simulink model "etb_positionControlModel"  (R2019b)
settings: Solver=FixedStepAuto  StartTime=0.0  StopTime=2  FixedStep=.001  RelTol=1e-3
values from neighbouring files (symbols this model uses):
  motorPosCmd = 60    [etb_positionControlModelSweep.m]
  motorPosGainI = 0    [etb_positionControlModelSweep.m]
  motorPosGainP = 1000:500:2500    [etb_positionControlModelSweep.m]
  motorVelGainFeedback = 200    [etb_positionControlModelSweep.m]
  motorVelGainI = 2500    [etb_positionControlModelSweep.m]
  motorVelGainP = 200:200:1000    [etb_positionControlModelSweep.m]
  springConst = 200    [etb_positionControlModelSweep.m]    (also in sweepSpringConstant.m = 300; sweepSpringFullSweep.m = 300; sweepSpringFullSweep_Ron.m = 300; sweepSpringPreload.m = 300)
  springPreload = 800    [etb_positionControlModelSweep.m]    (also in sweepSpringConstant.m = 780; sweepSpringFullSweep.m = 780; sweepSpringFullSweep_Ron.m = 780; sweepSpringPreload.m = 780)
undefined symbols (not defined in the file or in its folder): DiscIntNeverNeededParam
libraries: simulink x3, eeGeneralControl x1
settings Model: Creator=Nick  LastModifiedBy=Nick

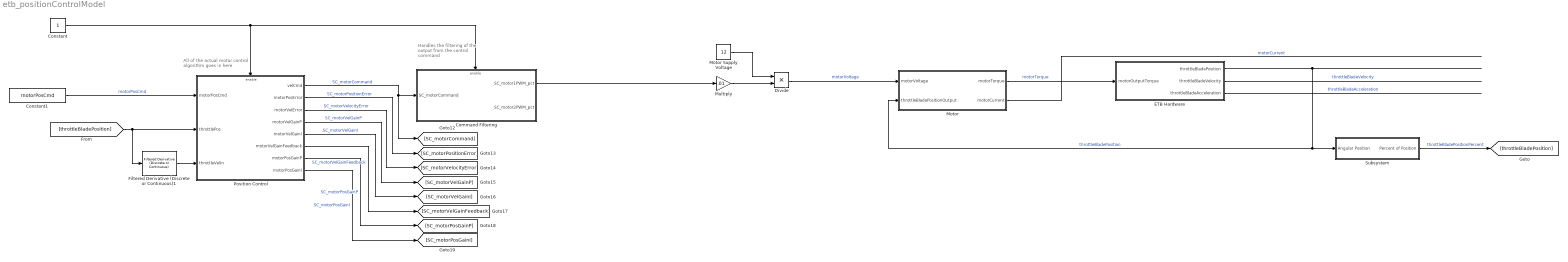
== system etb_positionControlModel ==
  note: All of the actual motor control algorithm goes in here
  note: Handles the filtering of the output from the control command
  Command Filtering : Subsystem
  Constant : Constant
  Constant1 : Constant  Value=motorPosCmd
  Divide : Product  Inputs=**
  ETB Hardware : Subsystem
  Filtered Derivative (Discrete or Continuous)1 : eeGeneralControl/Filtered Derivative (Discrete or Continuous)  K=1  T=0.01  B=inf  A=-inf  minRatio=10  Ts=-1
      settings: SourceProductName=Simscape Electrical  SourceProductBaseCode=PS
  Motor : Subsystem
  Motor Supply Voltage : Constant  Value=12
  Multiply : Gain  Gain=.01
  Position Control : Subsystem  TreatAsAtomicUnit=on
  Subsystem : Subsystem
  wires:
  ETB Hardware/2(throttleBladeVelocity) -> ?  "throttleBladeVelocity"
  ETB Hardware/3(throttleBladeAcceleration) -> ?  "throttleBladeAcceleration"
  Motor/1(motorTorque) -> ETB Hardware/1(motorOutputTorque)  "motorTorque"
  Motor/2(motorCurrent) -> ?  "motorCurrent"
  ETB Hardware/1(throttleBladePosition) -> Subsystem/1(Angular Position), Motor/2(throttleBladePositionOutput)  "throttleBladePosition"
  Divide/1 -> Motor/1(motorVoltage)  "motorVoltage"
  Multiply/1 -> Divide/2
  Motor Supply Voltage/1 -> Divide/1
  Command Filtering/1(SC_motor1PWM_pct) -> Multiply/1
  Subsystem/1(Percent of Position) -> [throttleBladePosition]  "throttleBladePositionPercent"
  [throttleBladePosition] -> Filtered Derivative (Discrete or Continuous)1/1, Position Control/2(throttlePos)
  Constant1/1 -> Position Control/1(motorPosCmd)  "motorPosCmd"
  Filtered Derivative (Discrete or Continuous)1/1 -> Position Control/3(throttleVelIn)
  Constant/1 -> Position Control/Enable, Command Filtering/Enable
  Position Control/1(velCmd) -> Command Filtering/1(SC_motorCommand), [SC_motorCommand]  "SC_motorCommand"
  Position Control/5(motorVelGainI) -> [SC_motorVelGainI]  "SC_motorVelGainI"
  Position Control/3(motorVelError) -> [SC_motorVelocityError]  "SC_motorVelocityError"
  Position Control/7(motorPosGainP) -> [SC_motorPosGainP]  "SC_motorPosGainP"
  Position Control/6(motorVelGainFeedback) -> [SC_motorVelGainFeedback]  "SC_motorVelGainFeedback"
  Position Control/4(motorVelGainP) -> [SC_motorVelGainP]  "SC_motorVelGainP"
  Position Control/2(motorPosError) -> [SC_motorPositionError]  "SC_motorPositionError"
  Position Control/8(motorPosGainI) -> [SC_motorPosGainI]  "SC_motorPosGainI"

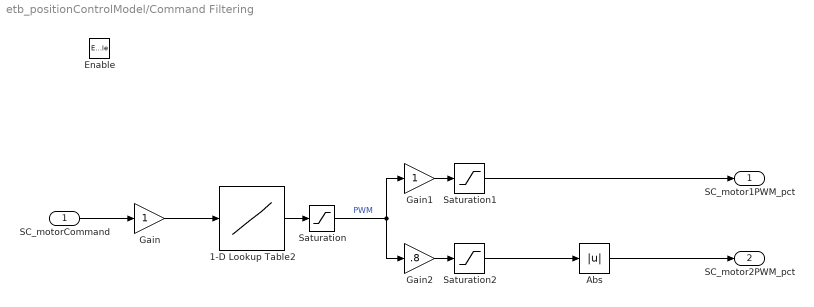
== system etb_positionControlModel/Command Filtering ==
  SC_motorCommand : Inport
  Enable : EnablePort  StatesWhenEnabling=reset
  1-D Lookup Table2 : Lookup_n-D  NumberOfTableDimensions=1  BreakpointsForDimension1=[-100 -5 -.1 0 .1 5 100]  Table=[-100 -5 -1 0 1 20 100]  InternalRulePriority=Speed  RndMeth=Simplest  InputSameDT=on
  Abs : Abs
  Gain : Gain
  Gain1 : Gain
  Gain2 : Gain  Gain=.8
  Saturation : Saturate  UpperLimit=100  LowerLimit=-100
  Saturation1 : Saturate  UpperLimit=100  LowerLimit=0
  Saturation2 : Saturate  UpperLimit=0  LowerLimit=-100
  SC_motor1PWM_pct : Outport
  SC_motor2PWM_pct : Outport  Port=2
  wires:
  Abs/1 -> SC_motor2PWM_pct/1
  1-D Lookup Table2/1 -> Saturation/1
  Gain/1 -> 1-D Lookup Table2/1
  Saturation2/1 -> Abs/1
  Gain1/1 -> Saturation1/1
  Gain2/1 -> Saturation2/1
  SC_motorCommand/1 -> Gain/1
  Saturation/1 -> Gain1/1, Gain2/1  "PWM"
  Saturation1/1 -> SC_motor1PWM_pct/1

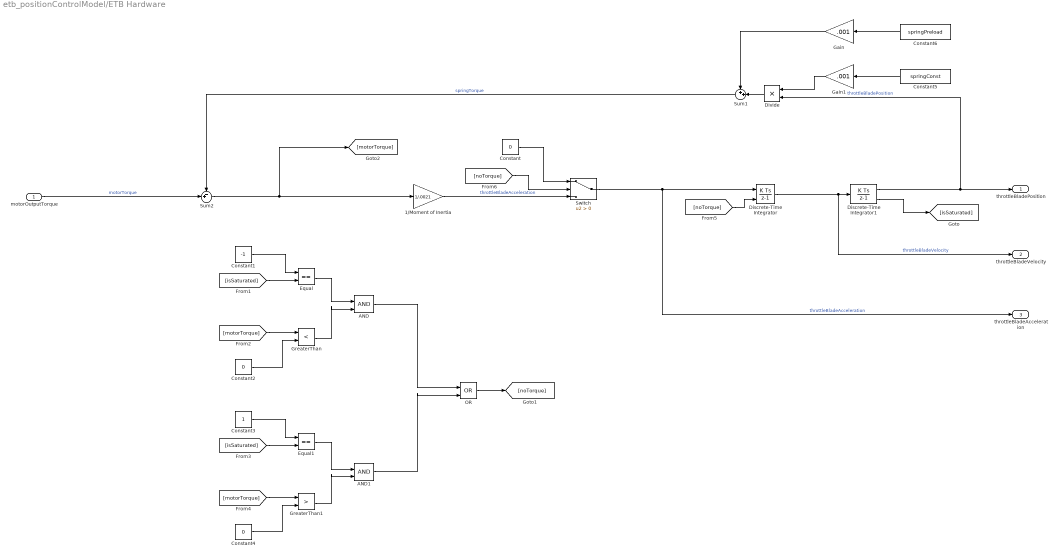
== system etb_positionControlModel/ETB Hardware ==
  motorOutputTorque : Inport
  1/Moment of Inertia : Gain  Gain=1/.0021
  AND : Logic  IconShape=distinctive  AllPortsSameDT=off  OutDataTypeStr=boolean
  AND1 : Logic  IconShape=distinctive  AllPortsSameDT=off  OutDataTypeStr=boolean
  Constant : Constant  Value=0
  Constant1 : Constant  Value=-1
  Constant2 : Constant  Value=0
  Constant3 : Constant
  Constant4 : Constant  Value=0
  Constant5 : Constant  Value=springConst
  Constant6 : Constant  Value=springPreload
  Discrete-Time Integrator : DiscreteIntegrator  ExternalReset=level  SampleTime=-1  ICPrevOutput=DiscIntNeverNeededParam  ICPrevScaledInput=DiscIntNeverNeededParam
  Discrete-Time Integrator1 : DiscreteIntegrator  SampleTime=-1  LimitOutput=on  UpperSaturationLimit=1.5708  LowerSaturationLimit=0  ShowSaturationPort=on  ICPrevOutput=DiscIntNeverNeededParam  ICPrevScaledInput=DiscIntNeverNeededParam
  Divide : Product  Inputs=**
  Equal : RelationalOperator  Operator===  OutDataTypeStr=boolean  RndMeth=Simplest
  Equal1 : RelationalOperator  Operator===  OutDataTypeStr=boolean  RndMeth=Simplest
  Gain : Gain  Gain=.001
  Gain1 : Gain  Gain=.001
  GreaterThan : RelationalOperator  Operator=<  OutDataTypeStr=boolean  RndMeth=Simplest
  GreaterThan1 : RelationalOperator  Operator=>  OutDataTypeStr=boolean  RndMeth=Simplest
  OR : Logic  Operator=OR  IconShape=distinctive  AllPortsSameDT=off  OutDataTypeStr=boolean
  Sum1 : Sum  Inputs=++|
  Sum2 : Sum  Inputs=-+|
  Switch : Switch  Criteria=u2 > Threshold
  throttleBladePosition : Outport
  throttleBladeVelocity : Outport  Port=2
  throttleBladeAcceleration : Outport  Port=3
  wires:
  Constant5/1 -> Gain1/1
  Gain1/1 -> Divide/1
  Constant6/1 -> Gain/1
  motorOutputTorque/1 -> Sum2/2  "motorTorque"
  Sum1/1 -> Sum2/1  "springTorque"
  Switch/1 -> Discrete-Time Integrator/1, throttleBladeAcceleration/1  "throttleBladeAcceleration"
  Discrete-Time Integrator/1 -> throttleBladeVelocity/1, Discrete-Time Integrator1/1  "throttleBladeVelocity"
  Discrete-Time Integrator1/1 -> throttleBladePosition/1, Divide/2  "throttleBladePosition"
  Divide/1 -> Sum1/2
  Gain/1 -> Sum1/1
  Sum2/1 -> 1/Moment of Inertia/1, [motorTorque]
  Constant1/1 -> Equal/1
  Equal/1 -> AND/1
  Discrete-Time Integrator1/2 -> [isSaturated]
  OR/1 -> [noTorque]
  [isSaturated] -> Equal/2
  GreaterThan/1 -> AND/2
  Constant2/1 -> GreaterThan/2
  [motorTorque] -> GreaterThan/1
  [motorTorque] -> GreaterThan1/1
  Constant4/1 -> GreaterThan1/2
  [isSaturated] -> Equal1/2
  Constant3/1 -> Equal1/1
  Equal1/1 -> AND1/1
  GreaterThan1/1 -> AND1/2
  AND/1 -> OR/1
  AND1/1 -> OR/2
  [noTorque] -> Discrete-Time Integrator/2
  1/Moment of Inertia/1 -> Switch/3  "throttleBladeAcceleration"
  [noTorque] -> Switch/2
  Constant/1 -> Switch/1

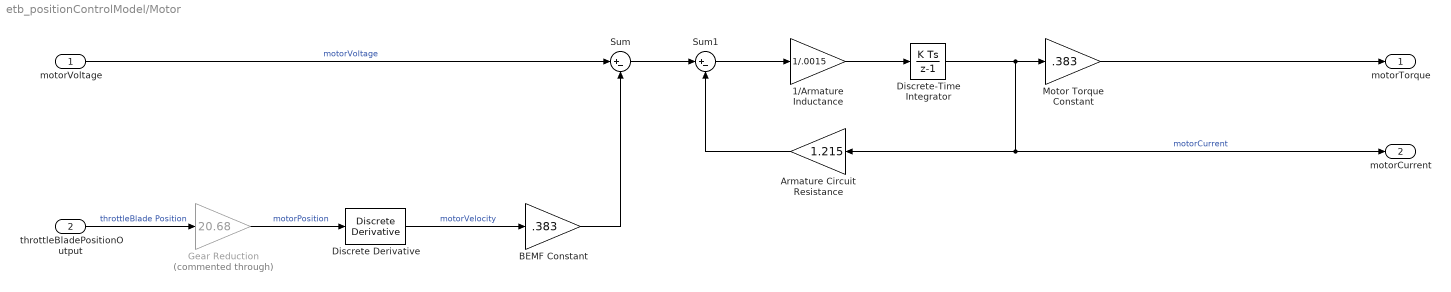
== system etb_positionControlModel/Motor ==
  motorVoltage : Inport
  throttleBladePositionOutput : Inport  Port=2
  1/Armature Inductance : Gain  Gain=1/.0015
  Armature Circuit Resistance : Gain  Gain=1.215
  BEMF Constant : Gain  Gain=.383
  Discrete Derivative : simulink/Discrete/Discrete Derivative  gainval=1.0  ICPrevScaledInput=0.0  OutMin=[]  OutMax=[]  OutDataType=fixdt(1, 16)  OutScaling=2^-10  DoSatur=off
  Discrete-Time Integrator : DiscreteIntegrator  SampleTime=-1  ICPrevOutput=DiscIntNeverNeededParam  ICPrevScaledInput=DiscIntNeverNeededParam
  Gear Reduction : Gain  Commented=through  Gain=20.68
  Motor Torque Constant : Gain  Gain=.383
  Sum : Sum  Inputs=|+-
  Sum1 : Sum  Inputs=|+-
  motorTorque : Outport
  motorCurrent : Outport  Port=2
  wires:
  Discrete-Time Integrator/1 -> Motor Torque Constant/1, motorCurrent/1, Armature Circuit Resistance/1  "motorCurrent"
  Motor Torque Constant/1 -> motorTorque/1
  motorVoltage/1 -> Sum/1  "motorVoltage"
  Armature Circuit Resistance/1 -> Sum1/2
  Sum1/1 -> 1/Armature Inductance/1
  1/Armature Inductance/1 -> Discrete-Time Integrator/1
  Sum/1 -> Sum1/1
  BEMF Constant/1 -> Sum/2
  throttleBladePositionOutput/1 -> Gear Reduction/1  "throttleBlade Position"
  Gear Reduction/1 -> Discrete Derivative/1  "motorPosition"
  Discrete Derivative/1 -> BEMF Constant/1  "motorVelocity"

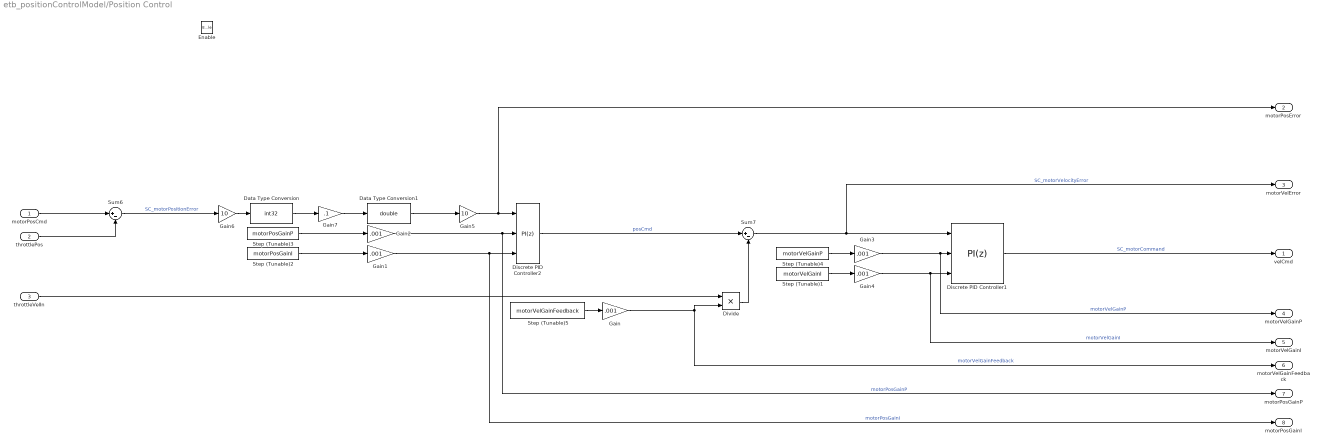
== system etb_positionControlModel/Position Control ==
  motorPosCmd : Inport
  throttlePos : Inport  Port=2
  throttleVelIn : Inport  Port=3
  Enable : EnablePort  StatesWhenEnabling=reset
  Data Type Conversion : DataTypeConversion  OutDataTypeStr=int32
  Data Type Conversion1 : DataTypeConversion  OutDataTypeStr=double
  Discrete PID Controller1 : simulink/Continuous/PID Controller  Controller=PI  Form=Ideal  TimeDomain=Discrete-time  SampleTime=-1  IntegratorMethod=Forward Euler  FilterMethod=Forward Euler  ControllerParametersSource=external  P=0  I=0  D=0  UseFilter=off  N=100  TunerSelectOption=Transfer Function Based (PID Tuner App)  InitialConditionSource=internal  InitialConditionForIntegrator=0  InitialConditionForFilter=0  DifferentiatorICPrevScaledInput=0  ExternalReset=none  TrackingMode=off  Kt=1  LimitOutput=on  UpperSaturationLimit=100  LowerSaturationLimit=-100  LinearizeAsGain=off  AntiWindupMode=none  Kb=1  POutMin=[]  POutMax=[]  IOutMin=[]  IOutMax=[]  DOutMin=[]  DOutMax=[]  NOutMin=[]  NOutMax=[]  SumOutMin=[]  SumOutMax=[]  SaturationOutMin=[]  SaturationOutMax=[]  PParamMin=[]  PParamMax=[]  IParamMin=[]  IParamMax=[]  DParamMin=[]  DParamMax=[]  NParamMin=[]  NParamMax=[]  KbParamMin=[]  KbParamMax=[]  KtParamMin=[]  KtParamMax=[]  KbOutMin=[]  KbOutMax=[]  KtOutMin=[]  KtOutMax=[]  IntegratorOutMin=[]  IntegratorOutMax=[]  FilterOutMin=[]  FilterOutMax=[]  SumI1OutMin=[]  SumI1OutMax=[]  SumI2OutMin=[]  SumI2OutMax=[]  SumI3OutMin=[]  SumI3OutMax=[]  SumI4OutMin=[]  SumI4OutMax=[]  SumDOutMin=[]  SumDOutMax=[]  DifferentiatorOutMin=[]  DifferentiatorOutMax=[]  FilterDiffOutCoefMin=[]  FilterDiffOutCoefMax=[]  ReciprocalOutMin=[]  ReciprocalOutMax=[]  SumDenOutMin=[]  SumDenOutMax=[]  SumNumOutMin=[]  SumNumOutMax=[]  DivideOutMin=[]  DivideOutMax=[]  IntegratorContinuousStateAttributes=''  IntegratorStateMustResolveToSignalObject=off  IntegratorRTWStateStorageClass=Auto  FilterContinuousStateAttributes=''  FilterStateMustResolveToSignalObject=off  FilterRTWStateStorageClass=Auto  ParallelPVariant=Passthrough  IdealPVariant=ExternalParameters  IVariant=ExternalParameters  DVariant=Disabled  IntegratorVariant=Discrete  SatVariant=Enabled  AWVariant=Passthrough  PCopyVariant=Disabled  TRVariant=Disabled  FdbkBlocksVariant=Forward  IdealPFdbkVariant=Disabled  SatFdbkVariant=Disabled  DerivativeFilterVariant=Disabled  NVariant=Disabled  NCopyVariant=Disabled_SignalSpec  FilterICVariant=Disabled  IntegratorICVariant=InternalICs  ExternalResetVariant=Disabled  TRSumVariant=Passthrough  SumFdbkVariant=Disabled  SumVariant=Sum_PI
  Discrete PID Controller2 : simulink/Continuous/PID Controller  Controller=PI  Form=Ideal  TimeDomain=Discrete-time  SampleTime=-1  IntegratorMethod=Forward Euler  FilterMethod=Forward Euler  ControllerParametersSource=external  P=0  I=0  D=0  UseFilter=off  N=100  TunerSelectOption=Transfer Function Based (PID Tuner App)  InitialConditionSource=internal  InitialConditionForIntegrator=0  InitialConditionForFilter=0  DifferentiatorICPrevScaledInput=0  ExternalReset=none  TrackingMode=off  Kt=1  LimitOutput=on  UpperSaturationLimit=500  LowerSaturationLimit=-500  LinearizeAsGain=off  AntiWindupMode=none  Kb=1  POutMin=[]  POutMax=[]  IOutMin=[]  IOutMax=[]  DOutMin=[]  DOutMax=[]  NOutMin=[]  NOutMax=[]  SumOutMin=[]  SumOutMax=[]  SaturationOutMin=[]  SaturationOutMax=[]  PParamMin=[]  PParamMax=[]  IParamMin=[]  IParamMax=[]  DParamMin=[]  DParamMax=[]  NParamMin=[]  NParamMax=[]  KbParamMin=[]  KbParamMax=[]  KtParamMin=[]  KtParamMax=[]  KbOutMin=[]  KbOutMax=[]  KtOutMin=[]  KtOutMax=[]  IntegratorOutMin=[]  IntegratorOutMax=[]  FilterOutMin=[]  FilterOutMax=[]  SumI1OutMin=[]  SumI1OutMax=[]  SumI2OutMin=[]  SumI2OutMax=[]  SumI3OutMin=[]  SumI3OutMax=[]  SumI4OutMin=[]  SumI4OutMax=[]  SumDOutMin=[]  SumDOutMax=[]  DifferentiatorOutMin=[]  DifferentiatorOutMax=[]  FilterDiffOutCoefMin=[]  FilterDiffOutCoefMax=[]  ReciprocalOutMin=[]  ReciprocalOutMax=[]  SumDenOutMin=[]  SumDenOutMax=[]  SumNumOutMin=[]  SumNumOutMax=[]  DivideOutMin=[]  DivideOutMax=[]  IntegratorContinuousStateAttributes=''  IntegratorStateMustResolveToSignalObject=off  IntegratorRTWStateStorageClass=Auto  FilterContinuousStateAttributes=''  FilterStateMustResolveToSignalObject=off  FilterRTWStateStorageClass=Auto  ParallelPVariant=Passthrough  IdealPVariant=ExternalParameters  IVariant=ExternalParameters  DVariant=Disabled  IntegratorVariant=Discrete  SatVariant=Enabled  AWVariant=Passthrough  PCopyVariant=Disabled  TRVariant=Disabled  FdbkBlocksVariant=Forward  IdealPFdbkVariant=Disabled  SatFdbkVariant=Disabled  DerivativeFilterVariant=Disabled  NVariant=Disabled  NCopyVariant=Disabled_SignalSpec  FilterICVariant=Disabled  IntegratorICVariant=InternalICs  ExternalResetVariant=Disabled  TRSumVariant=Passthrough  SumFdbkVariant=Disabled  SumVariant=Sum_PI
  Divide : Product  Inputs=**
  Gain{,1..4} (5 alike) : Gain  Gain=.001
  Gain5 : Gain  Gain=10
  Gain6 : Gain  Gain=10
  Gain7 : Gain  Gain=.1
  Step (Tunable)1 : Constant  Value=motorVelGainI  VectorParams1D=off  SampleTime=-1
  Step (Tunable)2 : Constant  Value=motorPosGainI  VectorParams1D=off  SampleTime=-1
  Step (Tunable)3 : Constant  Value=motorPosGainP  VectorParams1D=off  SampleTime=-1
  Step (Tunable)4 : Constant  Value=motorVelGainP  VectorParams1D=off  SampleTime=-1
  Step (Tunable)5 : Constant  Value=motorVelGainFeedback  VectorParams1D=off  SampleTime=-1
  Sum6 : Sum  Inputs=|+-
  Sum7 : Sum  Inputs=|+-
  velCmd : Outport
  motorPosError : Outport  Port=2
  motorVelError : Outport  Port=3
  motorVelGainP : Outport  Port=4
  motorVelGainI : Outport  Port=5
  motorVelGainFeedback : Outport  Port=6
  motorPosGainP : Outport  Port=7
  motorPosGainI : Outport  Port=8
  wires:
  Data Type Conversion1/1 -> Gain5/1
  Data Type Conversion/1 -> Gain7/1
  Gain7/1 -> Data Type Conversion1/1
  Gain6/1 -> Data Type Conversion/1
  Gain5/1 -> Discrete PID Controller2/1, motorPosError/1
  Gain4/1 -> Discrete PID Controller1/3, motorVelGainI/1  "motorVelGainI"
  Gain3/1 -> Discrete PID Controller1/2, motorVelGainP/1  "motorVelGainP"
  Gain2/1 -> Discrete PID Controller2/2, motorPosGainP/1  "motorPosGainP"
  Gain1/1 -> Discrete PID Controller2/3, motorPosGainI/1  "motorPosGainI"
  Gain/1 -> Divide/2, motorVelGainFeedback/1  "motorVelGainFeedback"
  Step (Tunable)5/1 -> Gain/1
  Discrete PID Controller2/1 -> Sum7/1  "posCmd"
  Step (Tunable)4/1 -> Gain3/1
  Sum7/1 -> motorVelError/1, Discrete PID Controller1/1  "SC_motorVelocityError"
  Discrete PID Controller1/1 -> velCmd/1  "SC_motorCommand"
  throttleVelIn/1 -> Divide/1
  Step (Tunable)1/1 -> Gain4/1
  Divide/1 -> Sum7/2
  throttlePos/1 -> Sum6/2
  Step (Tunable)2/1 -> Gain1/1
  Step (Tunable)3/1 -> Gain2/1
  motorPosCmd/1 -> Sum6/1
  Sum6/1 -> Gain6/1  "SC_motorPositionError"

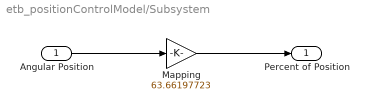
== system etb_positionControlModel/Subsystem ==
  Angular Position : Inport
  Mapping : Gain  Gain=63.66197723  OutMin=0  OutMax=100
  Percent of Position : Outport
  wires:
  Angular Position/1 -> Mapping/1
  Mapping/1 -> Percent of Position/1
